simulink model "AN_Simulink_Model_v1_fil"  (R2019b)
settings: Solver=VariableStepAuto  StartTime=0.0  StopTime=testtime  RelTol=1e-3
InitFcn:
  | AN_InitFcn_Callback
StopFcn:
  | AN_StopFcn_Callback
values from neighbouring files (symbols this model uses):
  tdres = 1/Fs    (= 2.08333333333e-05)    [AN_Set_Model_Parameters.m]
libraries: hdlmdlgenlib x163, simulink x4, fillib x1, dspsrcs4 x1
(part 2 of 5)

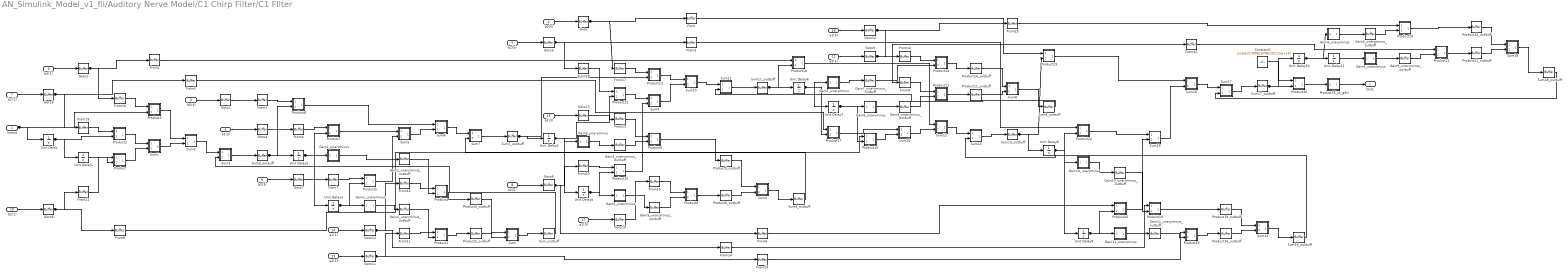
== system AN_Simulink_Model_v1_fil/Auditory Nerve Model/C1 Chirp Filter/C1 FIlter ==
  meout : Inport  OutDataTypeStr=single  PortDimensions=1  SampleTime=2.08333333333333e-05
  b0(5) : Inport  Port=2  OutDataTypeStr=single  PortDimensions=1  SampleTime=2.08333333333333e-05
  b0(3) : Inport  Port=3  OutDataTypeStr=single  PortDimensions=1  SampleTime=2.08333333333333e-05
  b0(1) : Inport  Port=4  OutDataTypeStr=single  PortDimensions=1  SampleTime=2.08333333333333e-05
  b1(5) : Inport  Port=5  OutDataTypeStr=single  PortDimensions=1  SampleTime=2.08333333333333e-05
  b1(3) : Inport  Port=6  OutDataTypeStr=single  PortDimensions=1  SampleTime=2.08333333333333e-05
  b1(1) : Inport  Port=7  OutDataTypeStr=single  PortDimensions=1  SampleTime=2.08333333333333e-05
  b2(5) : Inport  Port=8  OutDataTypeStr=single  PortDimensions=1  SampleTime=2.08333333333333e-05
  b2(3) : Inport  Port=9  OutDataTypeStr=single  PortDimensions=1  SampleTime=2.08333333333333e-05
  b2(1) : Inport  Port=10  OutDataTypeStr=single  PortDimensions=1  SampleTime=2.08333333333333e-05
  a2(5) : Inport  Port=11  OutDataTypeStr=single  PortDimensions=1  SampleTime=2.08333333333333e-05
  a2(3) : Inport  Port=12  OutDataTypeStr=single  PortDimensions=1  SampleTime=2.08333333333333e-05
  a2(1) : Inport  Port=13  OutDataTypeStr=single  PortDimensions=1  SampleTime=2.08333333333333e-05
  a1(1) : Inport  Port=14  OutDataTypeStr=single  PortDimensions=1  SampleTime=2.08333333333333e-05
  a1(3) : Inport  Port=15  OutDataTypeStr=single  PortDimensions=1  SampleTime=2.08333333333333e-05
  a1(5) : Inport  Port=16  OutDataTypeStr=single  PortDimensions=1  SampleTime=2.08333333333333e-05
  Constant1 : Constant  Value=single(3.398816786232115e+16)  OutDataTypeStr=single  SampleTime=-1
  From{,1..14,16..25} (25 alike) : hdlmdlgenlib/Buffer
      settings: SourceProductName=Simulink  SourceProductBaseCode=SL
  Gain10_unaryminus : Subsystem
      mask Display: disp('NFP\numinus');
  Gain10_unaryminus_outbuff : hdlmdlgenlib/Buffer
      settings: SourceProductName=Simulink  SourceProductBaseCode=SL
  Gain11_unaryminus : Subsystem
      mask Display: disp('NFP\numinus');
  Gain11_unaryminus_outbuff : hdlmdlgenlib/Buffer
      settings: SourceProductName=Simulink  SourceProductBaseCode=SL
  Gain1_unaryminus : Subsystem
      mask Display: disp('NFP\numinus');
  Gain1_unaryminus_outbuff : hdlmdlgenlib/Buffer
      settings: SourceProductName=Simulink  SourceProductBaseCode=SL
  Gain2_unaryminus : Subsystem
      mask Display: disp('NFP\numinus');
  Gain2_unaryminus_outbuff : hdlmdlgenlib/Buffer
      settings: SourceProductName=Simulink  SourceProductBaseCode=SL
  Gain3_unaryminus : Subsystem
      mask Display: disp('NFP\numinus');
  Gain3_unaryminus_outbuff : hdlmdlgenlib/Buffer
      settings: SourceProductName=Simulink  SourceProductBaseCode=SL
  Gain4_unaryminus : Subsystem
      mask Display: disp('NFP\numinus');
  Gain4_unaryminus_outbuff : hdlmdlgenlib/Buffer
      settings: SourceProductName=Simulink  SourceProductBaseCode=SL
  Gain5_unaryminus : Subsystem
      mask Display: disp('NFP\numinus');
  Gain5_unaryminus_outbuff : hdlmdlgenlib/Buffer
      settings: SourceProductName=Simulink  SourceProductBaseCode=SL
  Gain7_unaryminus : Subsystem
      mask Display: disp('NFP\numinus');
  Gain7_unaryminus_outbuff : hdlmdlgenlib/Buffer
      settings: SourceProductName=Simulink  SourceProductBaseCode=SL
  Gain8_unaryminus : Subsystem
      mask Display: disp('NFP\numinus');
  Gain8_unaryminus_outbuff : hdlmdlgenlib/Buffer
      settings: SourceProductName=Simulink  SourceProductBaseCode=SL
  Gain9_unaryminus : Subsystem
      mask Display: disp('NFP\numinus');
  Gain9_unaryminus_outbuff : hdlmdlgenlib/Buffer
      settings: SourceProductName=Simulink  SourceProductBaseCode=SL
  Goto{,1..14} (15 alike) : hdlmdlgenlib/Buffer
      settings: SourceProductName=Simulink  SourceProductBaseCode=SL
  Product : Subsystem
      mask Display: disp('NFP\nmul');
  Product1 : Subsystem
      mask Display: disp('NFP\nmul');
  Product10 : Subsystem
      mask Display: disp('NFP\nmul');
  Product11 : Subsystem
      mask Display: disp('NFP\nmul');
  Product11_outbuff : hdlmdlgenlib/Buffer
      settings: SourceProductName=Simulink  SourceProductBaseCode=SL
  Product12 : Subsystem
      mask Display: disp('NFP\nmul');
  Product13 : Subsystem
      mask Display: disp('NFP\nmul');
  Product14 : Subsystem
      mask Display: disp('NFP\nmul');
  Product14_outbuff : hdlmdlgenlib/Buffer
      settings: SourceProductName=Simulink  SourceProductBaseCode=SL
  Product15 : Subsystem
      mask Display: disp('NFP\nmul');
  Product16 : Subsystem
      mask Display: disp('NFP\nmul');
  Product16_outbuff : hdlmdlgenlib/Buffer
      settings: SourceProductName=Simulink  SourceProductBaseCode=SL
  Product17 : Subsystem
      mask Display: disp('NFP\nmul');
  Product18 : Subsystem
      mask Display: disp('NFP\nmul');
  Product19 : Subsystem
      mask Display: disp('NFP\nmul');
  Product19_outbuff : hdlmdlgenlib/Buffer
      settings: SourceProductName=Simulink  SourceProductBaseCode=SL
  Product1_outbuff : hdlmdlgenlib/Buffer
      settings: SourceProductName=Simulink  SourceProductBaseCode=SL
  Product2 : Subsystem
      mask Display: disp('NFP\nmul');
  Product20 : Subsystem
      mask Display: disp('NFP\nmul');
  Product21 : Subsystem
      mask Display: disp('NFP\nmul');
  Product21_outbuff : hdlmdlgenlib/Buffer
      settings: SourceProductName=Simulink  SourceProductBaseCode=SL
  Product22 : Subsystem
      mask Display: disp('NFP\nmul');
  Product23 : Subsystem
      mask Display: disp('NFP\nmul');
  Product24 : Subsystem
      mask Display: disp('NFP\nmul');
  Product24_outbuff : hdlmdlgenlib/Buffer
      settings: SourceProductName=Simulink  SourceProductBaseCode=SL
  Product25_to_gain : Subsystem
      mask Display: disp('NFP\ngain_pow2');
  Product26 : Subsystem
      mask Display: disp('NFP\nmul');
  Product3 : Subsystem
      mask Display: disp('NFP\nmul');
  Product4 : Subsystem
      mask Display: disp('NFP\nmul');
  Product4_outbuff : hdlmdlgenlib/Buffer
      settings: SourceProductName=Simulink  SourceProductBaseCode=SL
  Product5 : Subsystem
      mask Display: disp('NFP\nmul');
  Product6 : Subsystem
      mask Display: disp('NFP\nmul');
  Product6_outbuff : hdlmdlgenlib/Buffer
      settings: SourceProductName=Simulink  SourceProductBaseCode=SL
  Product7 : Subsystem
      mask Display: disp('NFP\nmul');
  Product8 : Subsystem
      mask Display: disp('NFP\nmul');
  Product9 : Subsystem
      mask Display: disp('NFP\nmul');
  Product9_outbuff : hdlmdlgenlib/Buffer
      settings: SourceProductName=Simulink  SourceProductBaseCode=SL
  Sum : Subsystem
      mask Display: disp('NFP\nadd');
  Sum1 : Subsystem
      mask Display: disp('NFP\nadd');
  Sum10 : Subsystem
      mask Display: disp('NFP\nadd');
  Sum11 : Subsystem
      mask Display: disp('NFP\nadd');
  Sum11_outbuff : hdlmdlgenlib/Buffer
      settings: SourceProductName=Simulink  SourceProductBaseCode=SL
  Sum12 : Subsystem
      mask Display: disp('NFP\nadd');
  Sum13 : Subsystem
      mask Display: disp('NFP\nadd');
  Sum13_outbuff : hdlmdlgenlib/Buffer
      settings: SourceProductName=Simulink  SourceProductBaseCode=SL
  Sum14 : Subsystem
      mask Display: disp('NFP\nadd');
  Sum14_outbuff : hdlmdlgenlib/Buffer
      settings: SourceProductName=Simulink  SourceProductBaseCode=SL
  Sum15 : Subsystem
      mask Display: disp('NFP\nadd');
  Sum16 : Subsystem
      mask Display: disp('NFP\nadd');
  Sum17 : Subsystem
      mask Display: disp('NFP\nadd');
  Sum17_outbuff : hdlmdlgenlib/Buffer
      settings: SourceProductName=Simulink  SourceProductBaseCode=SL
  Sum18 : Subsystem
      mask Display: disp('NFP\nadd');
  Sum18_outbuff : hdlmdlgenlib/Buffer
      settings: SourceProductName=Simulink  SourceProductBaseCode=SL
  Sum19 : Subsystem
      mask Display: disp('NFP\nadd');
  Sum2 : Subsystem
      mask Display: disp('NFP\nadd');
  Sum3 : Subsystem
      mask Display: disp('NFP\nadd');
  Sum3_outbuff : hdlmdlgenlib/Buffer
      settings: SourceProductName=Simulink  SourceProductBaseCode=SL
  Sum4 : Subsystem
      mask Display: disp('NFP\nadd');
  Sum4_outbuff : hdlmdlgenlib/Buffer
      settings: SourceProductName=Simulink  SourceProductBaseCode=SL
  Sum5 : Subsystem
      mask Display: disp('NFP\nadd');
  Sum6 : Subsystem
      mask Display: disp('NFP\nadd');
  Sum7 : Subsystem
      mask Display: disp('NFP\nadd');
  Sum7_outbuff : hdlmdlgenlib/Buffer
      settings: SourceProductName=Simulink  SourceProductBaseCode=SL
  Sum8 : Subsystem
      mask Display: disp('NFP\nadd');
  Sum8_outbuff : hdlmdlgenlib/Buffer
      settings: SourceProductName=Simulink  SourceProductBaseCode=SL
  Sum9 : Subsystem
      mask Display: disp('NFP\nadd');
  Sum_outbuff : hdlmdlgenlib/Buffer
      settings: SourceProductName=Simulink  SourceProductBaseCode=SL
  Unit Delay{,1..11} (12 alike) : UnitDelay  InitialCondition=single(0)  SampleTime=2.08333333333333e-05
  Out1 : Outport  VectorParamsAs1DForOutWhenUnconnected=off
  wires:
  Product25_to_gain/1(Out1) -> Out1/1
  Sum9/1(Out1) -> Sum10/2(In2)
  Sum8/1(Out1) -> Sum8_outbuff/1
  Sum7/1(Out1) -> Sum7_outbuff/1
  Sum6/1(Out1) -> Sum7/1(In1)
  Sum5/1(Out1) -> Sum6/2(In2)
  Sum4/1(Out1) -> Sum4_outbuff/1
  Sum3/1(Out1) -> Sum3_outbuff/1
  Sum2/1(Out1) -> Sum3/1(In1)
  Sum19/1(Out1) -> Sum16/2(In2)
  Sum18/1(Out1) -> Sum18_outbuff/1
  Sum17/1(Out1) -> Sum17_outbuff/1
  Sum16/1(Out1) -> Sum17/1(In1)
  Sum15/1(Out1) -> Sum12/2(In2)
  Sum14/1(Out1) -> Sum14_outbuff/1
  Sum13/1(Out1) -> Sum13_outbuff/1
  Sum12/1(Out1) -> Sum13/1(In1)
  Sum11/1(Out1) -> Sum11_outbuff/1
  Sum10/1(Out1) -> Sum11/1(In1)
  Sum1/1(Out1) -> Sum2/2(In2)
  Sum/1(Out1) -> Sum_outbuff/1
  Product9/1(Out1) -> Product9_outbuff/1
  Product8/1(Out1) -> Sum6/1(In1)
  Product7/1(Out1) -> Sum5/1(In1)
  Product6/1(Out1) -> Product6_outbuff/1
  Product5/1(Out1) -> Sum5/2(In2)
  Product4/1(Out1) -> Product4_outbuff/1
  Product3/1(Out1) -> Sum2/1(In1)
  Product26/1(Out1) -> Product25_to_gain/1(In1)
  Product24/1(Out1) -> Product24_outbuff/1
  Product23/1(Out1) -> Sum16/1(In1)
  Product22/1(Out1) -> Sum19/1(In1)
  Product21/1(Out1) -> Product21_outbuff/1
  Product20/1(Out1) -> Sum19/2(In2)
  Product2/1(Out1) -> Sum1/1(In1)
  Product19/1(Out1) -> Product19_outbuff/1
  Product18/1(Out1) -> Sum12/1(In1)
  Product17/1(Out1) -> Sum15/1(In1)
  Product16/1(Out1) -> Product16_outbuff/1
  Product15/1(Out1) -> Sum15/2(In2)
  Product14/1(Out1) -> Product14_outbuff/1
  Product13/1(Out1) -> Sum10/1(In1)
  Product12/1(Out1) -> Sum9/1(In1)
  Product11/1(Out1) -> Product11_outbuff/1
  Product10/1(Out1) -> Sum9/2(In2)
  Product1/1(Out1) -> Product1_outbuff/1
  Product/1(Out1) -> Sum1/2(In2)
  Gain9_unaryminus/1(Out1) -> Gain9_unaryminus_outbuff/1
  Gain8_unaryminus/1(Out1) -> Gain8_unaryminus_outbuff/1
  Gain7_unaryminus/1(Out1) -> Gain7_unaryminus_outbuff/1
  Gain5_unaryminus/1(Out1) -> Gain5_unaryminus_outbuff/1
  Gain4_unaryminus/1(Out1) -> Gain4_unaryminus_outbuff/1
  Gain3_unaryminus/1(Out1) -> Gain3_unaryminus_outbuff/1
  Gain2_unaryminus/1(Out1) -> Gain2_unaryminus_outbuff/1
  Gain11_unaryminus/1(Out1) -> Gain11_unaryminus_outbuff/1
  Gain10_unaryminus/1(Out1) -> Gain10_unaryminus_outbuff/1
  Gain1_unaryminus/1(Out1) -> Gain1_unaryminus_outbuff/1
  Goto7/1 -> From7/1
  Goto4/1 -> From4/1
  Goto9/1 -> From22/1, From9/1
  Goto8/1 -> From21/1, From8/1
  Goto6/1 -> From20/1, From6/1
  Goto5/1 -> From19/1, From5/1
  Goto3/1 -> From18/1, From3/1
  Goto2/1 -> From16/1, From2/1
  Goto14/1 -> From14/1, From25/1
  Goto13/1 -> From13/1
  Goto12/1 -> From12/1, From24/1
  Goto11/1 -> From11/1, From23/1
  Goto10/1 -> From10/1
  Goto1/1 -> From1/1
  Goto/1 -> From/1, From17/1
  Unit Delay9/1 -> Gain11_unaryminus/1(In1), Product20/2(In2)
  Unit Delay8/1 -> Unit Delay9/1, Gain10_unaryminus/1(In1), Product22/2(In2)
  Unit Delay7/1 -> Gain8_unaryminus/1(In1), Product15/2(In2)
  Unit Delay6/1 -> Unit Delay7/1, Gain7_unaryminus/1(In1), Product17/2(In2)
  Unit Delay5/1 -> Gain5_unaryminus/1(In1), Product10/2(In2)
  Unit Delay4/1 -> Unit Delay5/1, Gain3_unaryminus/1(In1), Product12/2(In2)
  Unit Delay3/1 -> Gain2_unaryminus/1(In1), Product5/2(In2)
  Unit Delay2/1 -> Unit Delay3/1, Gain1_unaryminus/1(In1), Product7/2(In2)
  Unit Delay11/1 -> Gain9_unaryminus/1(In1)
  Unit Delay10/1 -> Unit Delay11/1, Gain4_unaryminus/1(In1)
  Unit Delay1/1 -> Product/2(In2)
  Unit Delay/1 -> Unit Delay1/1, Product2/2(In2)
  Sum8_outbuff/1 -> Sum11/2(In2)
  Sum7_outbuff/1 -> Unit Delay4/1, Product13/2(In2)
  Sum4_outbuff/1 -> Sum7/2(In2)
  Sum3_outbuff/1 -> Unit Delay2/1, Product8/2(In2)
  Sum18_outbuff/1 -> Sum17/2(In2)
  Sum17_outbuff/1 -> Unit Delay10/1, Product26/2(In2)
  Sum14_outbuff/1 -> Sum13/2(In2)
  Sum13_outbuff/1 -> Unit Delay8/1, Product23/2(In2)
  Sum11_outbuff/1 -> Unit Delay6/1, Product18/2(In2)
  Sum_outbuff/1 -> Sum3/2(In2)
  Product9_outbuff/1 -> Sum4/1(In1)
  Product6_outbuff/1 -> Sum4/2(In2)
  Product4_outbuff/1 -> Sum/1(In1)
  Product24_outbuff/1 -> Sum18/1(In1)
  Product21_outbuff/1 -> Sum18/2(In2)
  Product19_outbuff/1 -> Sum14/1(In1)
  Product16_outbuff/1 -> Sum14/2(In2)
  Product14_outbuff/1 -> Sum8/1(In1)
  Product11_outbuff/1 -> Sum8/2(In2)
  Product1_outbuff/1 -> Sum/2(In2)
  Gain9_unaryminus_outbuff/1 -> Product21/2(In2)
  Gain8_unaryminus_outbuff/1 -> Product11/2(In2)
  Gain7_unaryminus_outbuff/1 -> Product14/2(In2)
  Gain5_unaryminus_outbuff/1 -> Product6/2(In2)
  Gain4_unaryminus_outbuff/1 -> Product24/2(In2)
  Gain3_unaryminus_outbuff/1 -> Product9/2(In2)
  Gain2_unaryminus_outbuff/1 -> Product1/2(In2)
  Gain11_unaryminus_outbuff/1 -> Product16/2(In2)
  Gain10_unaryminus_outbuff/1 -> Product19/2(In2)
  Gain1_unaryminus_outbuff/1 -> Product4/2(In2)
  From9/1 -> Product11/1(In1)
  From8/1 -> Product15/1(In1)
  From7/1 -> Product5/1(In1)
  From6/1 -> Product20/1(In1)
  From5/1 -> Product17/1(In1)
  From4/1 -> Product7/1(In1)
  From3/1 -> Product22/1(In1)
  From25/1 -> Product24/1(In1)
  From24/1 -> Product19/1(In1)
  From23/1 -> Product16/1(In1)
  From22/1 -> Product21/1(In1)
  From21/1 -> Product/1(In1)
  From20/1 -> Product10/1(In1)
  From2/1 -> Product18/1(In1)
  From19/1 -> Product2/1(In1)
  From18/1 -> Product12/1(In1)
  From17/1 -> Product13/1(In1)
  From16/1 -> Product3/1(In1)
  From14/1 -> Product14/1(In1)
  From13/1 -> Product9/1(In1)
  From12/1 -> Product4/1(In1)
  From11/1 -> Product1/1(In1)
  From10/1 -> Product6/1(In1)
  From1/1 -> Product8/1(In1)
  From/1 -> Product23/1(In1)
  Constant1/1 -> Product26/1(In1)
  a1(5)/1 -> Goto14/1
  a1(3)/1 -> Goto13/1
  a1(1)/1 -> Goto12/1
  a2(1)/1 -> Goto11/1
  a2(3)/1 -> Goto10/1
  a2(5)/1 -> Goto9/1
  b2(1)/1 -> Goto8/1
  b2(3)/1 -> Goto7/1
  b2(5)/1 -> Goto6/1
  b1(1)/1 -> Goto5/1
  b1(3)/1 -> Goto4/1
  b1(5)/1 -> Goto3/1
  b0(1)/1 -> Goto2/1
  b0(3)/1 -> Goto1/1
  b0(5)/1 -> Goto/1
  meout/1 -> Unit Delay/1, Product3/2(In2)

== system AN_Simulink_Model_v1_fil/Auditory Nerve Model/C1 Chirp Filter/Calculate C1filterout ==
  C1filterouttmp : Inport  OutDataTypeStr=single  PortDimensions=1  SampleTime=2.08333333333333e-05
  Gain1_unary : hdlmdlgenlib/Buffer
      settings: SourceProductName=Simulink  SourceProductBaseCode=SL
  C1filterout : Outport  VectorParamsAs1DForOutWhenUnconnected=off
  wires:
  Gain1_unary/1 -> C1filterout/1
  C1filterouttmp/1 -> Gain1_unary/1

== system AN_Simulink_Model_v1_fil/Auditory Nerve Model/C1 Chirp Filter/Calculate rsigma ==
  tauc1 : Inport  OutDataTypeStr=single  PortDimensions=1  SampleTime=2.08333333333333e-05
  Constant2 : Constant  Value=single(0.003011211520060897)  OutDataTypeStr=single  SampleTime=-1
  Reciprocal1_recip : Subsystem
      mask Display: disp('NFP\nmath');
  Reciprocal_recip : Subsystem
      mask Display: disp('NFP\nmath');
  Subtract : Subsystem
      mask Display: disp('NFP\nadd');
  rsigma : Outport  VectorParamsAs1DForOutWhenUnconnected=off
  wires:
  Subtract/1(Out1) -> rsigma/1
  Reciprocal1_recip/1(Out1) -> Subtract/2(In2)
  Reciprocal_recip/1(Out1) -> Subtract/1(In1)
  Constant2/1 -> Reciprocal1_recip/1(In1)
  tauc1/1 -> Reciprocal_recip/1(In1)

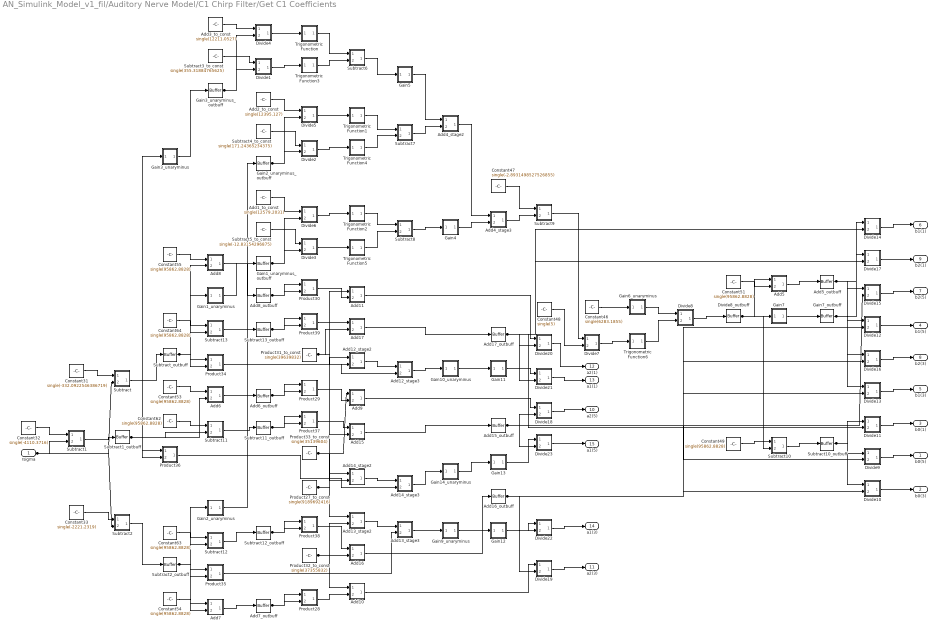
== system AN_Simulink_Model_v1_fil/Auditory Nerve Model/C1 Chirp Filter/Get C1 Coefficients ==
  rsigma : Inport  OutDataTypeStr=single  PortDimensions=1  SampleTime=2.08333333333333e-05
  Add10 : Subsystem
      mask Display: disp('NFP\nadd');
  Add11 : Subsystem
      mask Display: disp('NFP\nadd');
  Add12_stage2 : Subsystem
      mask Display: disp('NFP\nadd');
  Add12_stage3 : Subsystem
      mask Display: disp('NFP\nadd');
  Add13_stage2 : Subsystem
      mask Display: disp('NFP\nadd');
  Add13_stage3 : Subsystem
      mask Display: disp('NFP\nadd');
  Add14_stage2 : Subsystem
      mask Display: disp('NFP\nadd');
  Add14_stage3 : Subsystem
      mask Display: disp('NFP\nadd');
  Add15 : Subsystem
      mask Display: disp('NFP\nadd');
  Add15_outbuff : hdlmdlgenlib/Buffer
      settings: SourceProductName=Simulink  SourceProductBaseCode=SL
  Add16 : Subsystem
      mask Display: disp('NFP\nadd');
  Add16_outbuff : hdlmdlgenlib/Buffer
      settings: SourceProductName=Simulink  SourceProductBaseCode=SL
  Add17 : Subsystem
      mask Display: disp('NFP\nadd');
  Add17_outbuff : hdlmdlgenlib/Buffer
      settings: SourceProductName=Simulink  SourceProductBaseCode=SL
  Add1_to_const : Constant  Value=single(12579.2031)  OutDataTypeStr=single  SampleTime=-1
  Add2_to_const : Constant  Value=single(12395.127)  OutDataTypeStr=single  SampleTime=-1
  Add3_to_const : Constant  Value=single(12211.0527)  OutDataTypeStr=single  SampleTime=-1
  Add4_stage2 : Subsystem
      mask Display: disp('NFP\nadd');
  Add4_stage3 : Subsystem
      mask Display: disp('NFP\nadd');
  Add5 : Subsystem
      mask Display: disp('NFP\nadd');
  Add5_outbuff : hdlmdlgenlib/Buffer
      settings: SourceProductName=Simulink  SourceProductBaseCode=SL
  Add6 : Subsystem
      mask Display: disp('NFP\nadd');
  Add6_outbuff : hdlmdlgenlib/Buffer
      settings: SourceProductName=Simulink  SourceProductBaseCode=SL
  Add7 : Subsystem
      mask Display: disp('NFP\nadd');
  Add7_outbuff : hdlmdlgenlib/Buffer
      settings: SourceProductName=Simulink  SourceProductBaseCode=SL
  Add8 : Subsystem
      mask Display: disp('NFP\nadd');
  Add8_outbuff : hdlmdlgenlib/Buffer
      settings: SourceProductName=Simulink  SourceProductBaseCode=SL
  Add9 : Subsystem
      mask Display: disp('NFP\nadd');
  Constant31 : Constant  Value=single(-332.0922546386719)  OutDataTypeStr=single  SampleTime=-1
  Constant32 : Constant  Value=single(-4110.3716)  OutDataTypeStr=single  SampleTime=-1
  Constant33 : Constant  Value=single(-2221.2319)  OutDataTypeStr=single  SampleTime=-1
  Constant46 : Constant  Value=single(6283.1855)  OutDataTypeStr=single  SampleTime=-1
  Constant47 : Constant  Value=single(-2.8931498527526855)  OutDataTypeStr=single  SampleTime=-1
  Constant48 : Constant  Value=single(5)  OutDataTypeStr=single  SampleTime=-1
  Constant{49,51,53..55,62..64} (8 alike) : Constant  Value=single(95862.8828)  OutDataTypeStr=single  SampleTime=-1
  Divide1 : Subsystem
      mask Display: disp('NFP\nmul');
  Divide10 : Subsystem
      mask Display: disp('NFP\nmul');
  Divide11 : Subsystem
      mask Display: disp('NFP\nmul');
  Divide12 : Subsystem
      mask Display: disp('NFP\nmul');
  Divide13 : Subsystem
      mask Display: disp('NFP\nmul');
  Divide14 : Subsystem
      mask Display: disp('NFP\nmul');
  Divide15 : Subsystem
      mask Display: disp('NFP\nmul');
  Divide16 : Subsystem
      mask Display: disp('NFP\nmul');
  Divide17 : Subsystem
      mask Display: disp('NFP\nmul');
  Divide18 : Subsystem
      mask Display: disp('NFP\nmul');
  Divide19 : Subsystem
      mask Display: disp('NFP\nmul');
  Divide2 : Subsystem
      mask Display: disp('NFP\nmul');
  Divide20 : Subsystem
      mask Display: disp('NFP\nmul');
  Divide21 : Subsystem
      mask Display: disp('NFP\nmul');
  Divide22 : Subsystem
      mask Display: disp('NFP\nmul');
  Divide23 : Subsystem
      mask Display: disp('NFP\nmul');
  Divide3 : Subsystem
      mask Display: disp('NFP\nmul');
  Divide4 : Subsystem
      mask Display: disp('NFP\nmul');
  Divide5 : Subsystem
      mask Display: disp('NFP\nmul');
  Divide6 : Subsystem
      mask Display: disp('NFP\nmul');
  Divide7 : Subsystem
      mask Display: disp('NFP\nmul');
  Divide8 : Subsystem
      mask Display: disp('NFP\nmul');
  Divide8_outbuff : hdlmdlgenlib/Buffer
      settings: SourceProductName=Simulink  SourceProductBaseCode=SL
  Divide9 : Subsystem
      mask Display: disp('NFP\nmul');
  Gain10_unaryminus : Subsystem
      mask Display: disp('NFP\numinus');
  Gain11 : Subsystem
      mask Display: disp('NFP\ngain_pow2');
  Gain12 : Subsystem
      mask Display: disp('NFP\ngain_pow2');
  Gain13 : Subsystem
      mask Display: disp('NFP\ngain_pow2');
  Gain14_unaryminus : Subsystem
      mask Display: disp('NFP\numinus');
  Gain1_unaryminus : Subsystem
      mask Display: disp('NFP\numinus');
  Gain1_unaryminus_outbuff : hdlmdlgenlib/Buffer
      settings: SourceProductName=Simulink  SourceProductBaseCode=SL
  Gain2_unaryminus : Subsystem
      mask Display: disp('NFP\numinus');
  Gain2_unaryminus_outbuff : hdlmdlgenlib/Buffer
      settings: SourceProductName=Simulink  SourceProductBaseCode=SL
  Gain3_unaryminus : Subsystem
      mask Display: disp('NFP\numinus');
  Gain3_unaryminus_outbuff : hdlmdlgenlib/Buffer
      settings: SourceProductName=Simulink  SourceProductBaseCode=SL
  Gain4 : Subsystem
      mask Display: disp('NFP\ngain_pow2');
  Gain5 : Subsystem
      mask Display: disp('NFP\ngain_pow2');
  Gain6_unaryminus : Subsystem
      mask Display: disp('NFP\numinus');
  Gain7 : Subsystem
      mask Display: disp('NFP\ngain_pow2');
  Gain7_outbuff : hdlmdlgenlib/Buffer
      settings: SourceProductName=Simulink  SourceProductBaseCode=SL
  Gain9_unaryminus : Subsystem
      mask Display: disp('NFP\numinus');
  Product27_to_const : Constant  Value=single(9189692416)  OutDataTypeStr=single  SampleTime=-1
  Product28 : Subsystem
      mask Display: disp('NFP\nmul');
  Product29 : Subsystem
      mask Display: disp('NFP\nmul');
  Product30 : Subsystem
      mask Display: disp('NFP\nmul');
  Product31_to_const : Constant  Value=single(39639832)  OutDataTypeStr=single  SampleTime=-1
  Product32_to_const : Constant  Value=single(37355832)  OutDataTypeStr=single  SampleTime=-1
  Product33_to_const : Constant  Value=single(35139604)  OutDataTypeStr=single  SampleTime=-1
  Product34 : Subsystem
      mask Display: disp('NFP\nmul');
  Product35 : Subsystem
      mask Display: disp('NFP\nmul');
  Product36 : Subsystem
      mask Display: disp('NFP\nmul');
  Product37 : Subsystem
      mask Display: disp('NFP\nmul');
  Product38 : Subsystem
      mask Display: disp('NFP\nmul');
  Product39 : Subsystem
      mask Display: disp('NFP\nmul');
  Subtract : Subsystem
      mask Display: disp('NFP\nadd');
  Subtract1 : Subsystem
      mask Display: disp('NFP\nadd');
  Subtract10 : Subsystem
      mask Display: disp('NFP\nadd');
  Subtract10_outbuff : hdlmdlgenlib/Buffer
      settings: SourceProductName=Simulink  SourceProductBaseCode=SL
  Subtract11 : Subsystem
      mask Display: disp('NFP\nadd');
  Subtract11_outbuff : hdlmdlgenlib/Buffer
      settings: SourceProductName=Simulink  SourceProductBaseCode=SL
  Subtract12 : Subsystem
      mask Display: disp('NFP\nadd');
  Subtract12_outbuff : hdlmdlgenlib/Buffer
      settings: SourceProductName=Simulink  SourceProductBaseCode=SL
  Subtract13 : Subsystem
      mask Display: disp('NFP\nadd');
  Subtract13_outbuff : hdlmdlgenlib/Buffer
      settings: SourceProductName=Simulink  SourceProductBaseCode=SL
  Subtract1_outbuff : hdlmdlgenlib/Buffer
      settings: SourceProductName=Simulink  SourceProductBaseCode=SL
  Subtract2 : Subsystem
      mask Display: disp('NFP\nadd');
  Subtract2_outbuff : hdlmdlgenlib/Buffer
      settings: SourceProductName=Simulink  SourceProductBaseCode=SL
  Subtract3_to_const : Constant  Value=single(355.31884765625)  OutDataTypeStr=single  SampleTime=-1
  Subtract4_to_const : Constant  Value=single(171.24365234375)  OutDataTypeStr=single  SampleTime=-1
  Subtract5_to_const : Constant  Value=single(-12.83154296875)  OutDataTypeStr=single  SampleTime=-1
  Subtract6 : Subsystem
      mask Display: disp('NFP\nadd');
  Subtract7 : Subsystem
      mask Display: disp('NFP\nadd');
  Subtract8 : Subsystem
      mask Display: disp('NFP\nadd');
  Subtract9 : Subsystem
      mask Display: disp('NFP\nadd');
  Subtract_outbuff : hdlmdlgenlib/Buffer
      settings: SourceProductName=Simulink  SourceProductBaseCode=SL
  Trigonometric Function : Subsystem
      mask Display: disp('NFP\ntrig');
  Trigonometric Function1 : Subsystem
      mask Display: disp('NFP\ntrig');
  Trigonometric Function2 : Subsystem
      mask Display: disp('NFP\ntrig');
  Trigonometric Function3 : Subsystem
      mask Display: disp('NFP\ntrig');
  Trigonometric Function4 : Subsystem
      mask Display: disp('NFP\ntrig');
  Trigonometric Function5 : Subsystem
      mask Display: disp('NFP\ntrig');
  Trigonometric Function6 : Subsystem
      mask Display: disp('NFP\ntrig');
  b0(5) : Outport  VectorParamsAs1DForOutWhenUnconnected=off
  b0(3) : Outport  Port=2  VectorParamsAs1DForOutWhenUnconnected=off
  b0(1) : Outport  Port=3  VectorParamsAs1DForOutWhenUnconnected=off
  b1(5) : Outport  Port=4  VectorParamsAs1DForOutWhenUnconnected=off
  b1(3) : Outport  Port=5  VectorParamsAs1DForOutWhenUnconnected=off
  b1(1) : Outport  Port=6  VectorParamsAs1DForOutWhenUnconnected=off
  b2(5) : Outport  Port=7  VectorParamsAs1DForOutWhenUnconnected=off
  b2(3) : Outport  Port=8  VectorParamsAs1DForOutWhenUnconnected=off
  b2(1) : Outport  Port=9  VectorParamsAs1DForOutWhenUnconnected=off
  a2(5) : Outport  Port=10  VectorParamsAs1DForOutWhenUnconnected=off
  a2(3) : Outport  Port=11  VectorParamsAs1DForOutWhenUnconnected=off
  a2(1) : Outport  Port=12  VectorParamsAs1DForOutWhenUnconnected=off
  a1(1) : Outport  Port=13  VectorParamsAs1DForOutWhenUnconnected=off
  a1(3) : Outport  Port=14  VectorParamsAs1DForOutWhenUnconnected=off
  a1(5) : Outport  Port=15  VectorParamsAs1DForOutWhenUnconnected=off
  wires:
  Trigonometric Function6/1(Out1) -> Divide8/2(In2)
  Trigonometric Function5/1(Out1) -> Subtract8/2(In2)
  Trigonometric Function4/1(Out1) -> Subtract7/2(In2)
  Trigonometric Function3/1(Out1) -> Subtract6/2(In2)
  Trigonometric Function2/1(Out1) -> Subtract8/1(In1)
  Trigonometric Function1/1(Out1) -> Subtract7/1(In1)
  Trigonometric Function/1(Out1) -> Subtract6/1(In1)
  Subtract9/1(Out1) -> Divide7/1(In1)
  Subtract8/1(Out1) -> Gain4/1(In1)
  Subtract7/1(Out1) -> Add4_stage2/2(In2)
  Subtract6/1(Out1) -> Gain5/1(In1)
  Subtract2/1(Out1) -> Subtract2_outbuff/1
  Subtract13/1(Out1) -> Subtract13_outbuff/1
  Subtract12/1(Out1) -> Subtract12_outbuff/1
  Subtract11/1(Out1) -> Subtract11_outbuff/1
  Subtract10/1(Out1) -> Subtract10_outbuff/1
  Subtract1/1(Out1) -> Subtract1_outbuff/1
  Subtract/1(Out1) -> Subtract_outbuff/1
  Product39/1(Out1) -> Add17/1(In1)
  Product38/1(Out1) -> Add16/1(In1)
  Product37/1(Out1) -> Add15/1(In1)
  Product36/1(Out1) -> Add14_stage3/2(In2)
  Product35/1(Out1) -> Add13_stage3/2(In2)
  Product34/1(Out1) -> Add12_stage3/2(In2)
  Product30/1(Out1) -> Add11/2(In2)
  Product29/1(Out1) -> Add9/2(In2)
  Product28/1(Out1) -> Add10/2(In2)
  Divide9/1(Out1) -> b0(5)/1
  Divide8/1(Out1) -> Divide8_outbuff/1
  Divide7/1(Out1) -> Trigonometric Function6/1(In1)
  Divide6/1(Out1) -> Trigonometric Function2/1(In1)
  Divide5/1(Out1) -> Trigonometric Function1/1(In1)
  Divide4/1(Out1) -> Trigonometric Function/1(In1)
  Divide3/1(Out1) -> Trigonometric Function5/1(In1)
  Divide23/1(Out1) -> a1(5)/1
  Divide22/1(Out1) -> a1(3)/1
  Divide21/1(Out1) -> a1(1)/1
  Divide20/1(Out1) -> a2(1)/1
  Divide2/1(Out1) -> Trigonometric Function4/1(In1)
  Divide19/1(Out1) -> a2(3)/1
  Divide18/1(Out1) -> a2(5)/1
  Divide17/1(Out1) -> b2(1)/1
  Divide16/1(Out1) -> b2(3)/1
  Divide15/1(Out1) -> b2(5)/1
  Divide14/1(Out1) -> b1(1)/1
  Divide13/1(Out1) -> b1(3)/1
  Divide12/1(Out1) -> b1(5)/1
  Divide11/1(Out1) -> b0(1)/1
  Divide10/1(Out1) -> b0(3)/1
  Divide1/1(Out1) -> Trigonometric Function3/1(In1)
  Add9/1(Out1) -> Divide18/1(In1)
  Add8/1(Out1) -> Add8_outbuff/1
  Add7/1(Out1) -> Add7_outbuff/1
  Add6/1(Out1) -> Add6_outbuff/1
  Add5/1(Out1) -> Add5_outbuff/1
  Add4_stage3/1(Out1) -> Subtract9/2(In2)
  Add4_stage2/1(Out1) -> Add4_stage3/1(In1)
  Add17/1(Out1) -> Add17_outbuff/1
  Add16/1(Out1) -> Add16_outbuff/1
  Add15/1(Out1) -> Add15_outbuff/1
  Add14_stage3/1(Out1) -> Gain14_unaryminus/1(In1)
  Add14_stage2/1(Out1) -> Add14_stage3/1(In1)
  Add13_stage3/1(Out1) -> Gain9_unaryminus/1(In1)
  Add13_stage2/1(Out1) -> Add13_stage3/1(In1)
  Add12_stage3/1(Out1) -> Gain10_unaryminus/1(In1)
  Add12_stage2/1(Out1) -> Add12_stage3/1(In1)
  Add11/1(Out1) -> Divide20/1(In1)
  Add10/1(Out1) -> Divide19/1(In1)
  Gain9_unaryminus/1(Out1) -> Gain12/1(In1)
  Gain7/1(Out1) -> Gain7_outbuff/1
  Gain6_unaryminus/1(Out1) -> Divide8/1(In1)
  Gain5/1(Out1) -> Add4_stage2/1(In1)
  Gain4/1(Out1) -> Add4_stage3/2(In2)
  Gain3_unaryminus/1(Out1) -> Gain3_unaryminus_outbuff/1
  Gain2_unaryminus/1(Out1) -> Gain2_unaryminus_outbuff/1
  Gain14_unaryminus/1(Out1) -> Gain13/1(In1)
  Gain13/1(Out1) -> Divide23/1(In1)
  Gain12/1(Out1) -> Divide22/1(In1)
  Gain11/1(Out1) -> Divide21/1(In1)
  Gain10_unaryminus/1(Out1) -> Gain11/1(In1)
  Gain1_unaryminus/1(Out1) -> Gain1_unaryminus_outbuff/1
  Subtract5_to_const/1 -> Divide3/1(In1)
  Subtract4_to_const/1 -> Divide2/1(In1)
  Subtract3_to_const/1 -> Divide1/1(In1)
  Subtract2_outbuff/1 -> Gain2_unaryminus/1(In1), Add7/2(In2), Product35/1(In1), Product35/2(In2), Subtract12/2(In2)
  Subtract13_outbuff/1 -> Product39/1(In1), Product39/2(In2)
  Subtract12_outbuff/1 -> Product38/1(In1), Product38/2(In2)
  Subtract11_outbuff/1 -> Product37/1(In1), Product37/2(In2)
  Subtract10_outbuff/1 -> Divide10/1(In1), Divide11/1(In1), Divide9/1(In1)
  Subtract1_outbuff/1 -> Gain3_unaryminus/1(In1), Add6/2(In2), Product36/1(In1), Product36/2(In2), Subtract11/2(In2)
  Subtract_outbuff/1 -> Gain1_unaryminus/1(In1), Add8/2(In2), Product34/1(In1), Product34/2(In2), Subtract13/2(In2)
  Product33_to_const/1 -> Add14_stage2/2(In2), Add15/2(In2), Add9/1(In1)
  Product32_to_const/1 -> Add10/1(In1), Add13_stage2/2(In2), Add16/2(In2)
  Product31_to_const/1 -> Add11/1(In1), Add12_stage2/2(In2), Add17/2(In2)
  Product27_to_const/1 -> Add12_stage2/1(In1), Add13_stage2/1(In1), Add14_stage2/1(In1)
  Gain7_outbuff/1 -> Divide12/1(In1), Divide13/1(In1), Divide14/1(In1)
  Gain3_unaryminus_outbuff/1 -> Divide1/2(In2), Divide4/2(In2)
  Gain2_unaryminus_outbuff/1 -> Divide2/2(In2), Divide5/2(In2)
  Gain1_unaryminus_outbuff/1 -> Divide3/2(In2), Divide6/2(In2)
  Divide8_outbuff/1 -> Gain7/1(In1), Add5/1(In1), Subtract10/2(In2)
  Constant64/1 -> Subtract13/1(In1)
  Constant63/1 -> Subtract12/1(In1)
  Constant62/1 -> Subtract11/1(In1)
  Constant55/1 -> Add8/1(In1)
  Constant54/1 -> Add7/1(In1)
  Constant53/1 -> Add6/1(In1)
  Constant51/1 -> Add5/2(In2)
  Constant49/1 -> Subtract10/1(In1)
  Constant48/1 -> Divide7/2(In2)
  Constant47/1 -> Subtract9/1(In1)
  Constant46/1 -> Gain6_unaryminus/1(In1)
  Constant33/1 -> Subtract2/1(In1)
  Constant32/1 -> Subtract1/1(In1)
  Constant31/1 -> Subtract/1(In1)
  Add8_outbuff/1 -> Product30/1(In1), Product30/2(In2)
  Add7_outbuff/1 -> Product28/1(In1), Product28/2(In2)
  Add6_outbuff/1 -> Product29/1(In1), Product29/2(In2)
  Add5_outbuff/1 -> Divide15/1(In1), Divide16/1(In1), Divide17/1(In1)
  Add3_to_const/1 -> Divide4/1(In1)
  Add2_to_const/1 -> Divide5/1(In1)
  Add17_outbuff/1 -> Divide11/2(In2), Divide14/2(In2), Divide17/2(In2), Divide20/2(In2), Divide21/2(In2)
  Add16_outbuff/1 -> Divide10/2(In2), Divide13/2(In2), Divide16/2(In2), Divide19/2(In2), Divide22/2(In2)
  Add15_outbuff/1 -> Divide12/2(In2), Divide15/2(In2), Divide18/2(In2), Divide23/2(In2), Divide9/2(In2)
  Add1_to_const/1 -> Divide6/1(In1)
  rsigma/1 -> Subtract/2(In2), Subtract1/2(In2), Subtract2/2(In2)

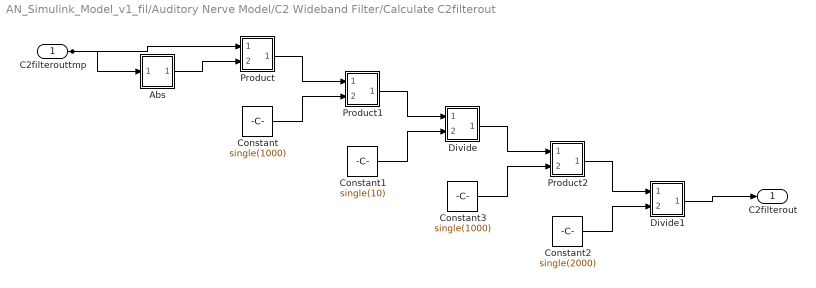
== system AN_Simulink_Model_v1_fil/Auditory Nerve Model/C2 Wideband Filter/Calculate C2filterout ==
  C2filterouttmp : Inport  OutDataTypeStr=single  PortDimensions=1  SampleTime=2.08333333333333e-05
  Abs : Subsystem
      mask Display: disp('NFP\nabs');
  Constant : Constant  Value=single(1000)  OutDataTypeStr=single  SampleTime=-1
  Constant1 : Constant  Value=single(10)  OutDataTypeStr=single  SampleTime=-1
  Constant2 : Constant  Value=single(2000)  OutDataTypeStr=single  SampleTime=-1
  Constant3 : Constant  Value=single(1000)  OutDataTypeStr=single  SampleTime=-1
  Divide : Subsystem
      mask Display: disp('NFP\nmul');
  Divide1 : Subsystem
      mask Display: disp('NFP\nmul');
  Product : Subsystem
      mask Display: disp('NFP\nmul');
  Product1 : Subsystem
      mask Display: disp('NFP\nmul');
  Product2 : Subsystem
      mask Display: disp('NFP\nmul');
  C2filterout : Outport  VectorParamsAs1DForOutWhenUnconnected=off
  wires:
  Product2/1(Out1) -> Divide1/1(In1)
  Product1/1(Out1) -> Divide/1(In1)
  Product/1(Out1) -> Product1/1(In1)
  Divide1/1(Out1) -> C2filterout/1
  Divide/1(Out1) -> Product2/1(In1)
  Abs/1(Out1) -> Product/2(In2)
  Constant3/1 -> Product2/2(In2)
  Constant2/1 -> Divide1/2(In2)
  Constant1/1 -> Divide/2(In2)
  Constant/1 -> Product1/2(In2)
  C2filterouttmp/1 -> Abs/1(In1), Product/1(In1)

== system AN_Simulink_Model_v1_fil/Auditory Nerve Model/C2 Wideband Filter/Gain ==
  In1 : Inport
  In2 : Inport  Port=2
  Gain : Product  Inputs=**  OutDataTypeStr=single  SampleTime=2.08333333333333e-05
  Out1 : Outport
  wires:
  Gain/1 -> Out1/1
  In2/1 -> Gain/2
  In1/1 -> Gain/1

== system AN_Simulink_Model_v1_fil/Auditory Nerve Model/C2 Wideband Filter/Gain10_unaryminus ==
  In1 : Inport
  Gain10_unaryminus : UnaryMinus  SampleTime=2.08333333333333e-05
  Out1 : Outport
  wires:
  Gain10_unaryminus/1 -> Out1/1
  In1/1 -> Gain10_unaryminus/1

== system AN_Simulink_Model_v1_fil/Auditory Nerve Model/C2 Wideband Filter/Gain1_unaryminus ==
  In1 : Inport
  Gain1_unaryminus : UnaryMinus  SampleTime=2.08333333333333e-05
  Out1 : Outport
  wires:
  Gain1_unaryminus/1 -> Out1/1
  In1/1 -> Gain1_unaryminus/1

== system AN_Simulink_Model_v1_fil/Auditory Nerve Model/C2 Wideband Filter/Gain2_unaryminus ==
  In1 : Inport
  Gain2_unaryminus : UnaryMinus  SampleTime=2.08333333333333e-05
  Out1 : Outport
  wires:
  Gain2_unaryminus/1 -> Out1/1
  In1/1 -> Gain2_unaryminus/1

== system AN_Simulink_Model_v1_fil/Auditory Nerve Model/C2 Wideband Filter/Gain3_unaryminus ==
  In1 : Inport
  Gain3_unaryminus : UnaryMinus  SampleTime=2.08333333333333e-05
  Out1 : Outport
  wires:
  Gain3_unaryminus/1 -> Out1/1
  In1/1 -> Gain3_unaryminus/1

== system AN_Simulink_Model_v1_fil/Auditory Nerve Model/C2 Wideband Filter/Gain4_unaryminus ==
  In1 : Inport
  Gain4_unaryminus : UnaryMinus  SampleTime=2.08333333333333e-05
  Out1 : Outport
  wires:
  Gain4_unaryminus/1 -> Out1/1
  In1/1 -> Gain4_unaryminus/1

== system AN_Simulink_Model_v1_fil/Auditory Nerve Model/C2 Wideband Filter/Gain5_unaryminus ==
  In1 : Inport
  Gain5_unaryminus : UnaryMinus  SampleTime=2.08333333333333e-05
  Out1 : Outport
  wires:
  Gain5_unaryminus/1 -> Out1/1
  In1/1 -> Gain5_unaryminus/1

== system AN_Simulink_Model_v1_fil/Auditory Nerve Model/C2 Wideband Filter/Gain6_unaryminus ==
  In1 : Inport
  Gain6_unaryminus : UnaryMinus  SampleTime=2.08333333333333e-05
  Out1 : Outport
  wires:
  Gain6_unaryminus/1 -> Out1/1
  In1/1 -> Gain6_unaryminus/1

== system AN_Simulink_Model_v1_fil/Auditory Nerve Model/C2 Wideband Filter/Gain7_unaryminus ==
  In1 : Inport
  Gain7_unaryminus : UnaryMinus  SampleTime=2.08333333333333e-05
  Out1 : Outport
  wires:
  Gain7_unaryminus/1 -> Out1/1
  In1/1 -> Gain7_unaryminus/1

== system AN_Simulink_Model_v1_fil/Auditory Nerve Model/C2 Wideband Filter/Gain8_unaryminus ==
  In1 : Inport
  Gain8_unaryminus : UnaryMinus  SampleTime=2.08333333333333e-05
  Out1 : Outport
  wires:
  Gain8_unaryminus/1 -> Out1/1
  In1/1 -> Gain8_unaryminus/1

== system AN_Simulink_Model_v1_fil/Auditory Nerve Model/C2 Wideband Filter/Gain9_unaryminus ==
  In1 : Inport
  Gain9_unaryminus : UnaryMinus  SampleTime=2.08333333333333e-05
  Out1 : Outport
  wires:
  Gain9_unaryminus/1 -> Out1/1
  In1/1 -> Gain9_unaryminus/1

== system AN_Simulink_Model_v1_fil/Auditory Nerve Model/C2 Wideband Filter/Product ==
  In1 : Inport
  In2 : Inport  Port=2
  Product : Product  Inputs=**  OutDataTypeStr=single  SampleTime=2.08333333333333e-05
  Out1 : Outport
  wires:
  Product/1 -> Out1/1
  In2/1 -> Product/2
  In1/1 -> Product/1

== system AN_Simulink_Model_v1_fil/Auditory Nerve Model/C2 Wideband Filter/Product1 ==
  In1 : Inport
  In2 : Inport  Port=2
  Product1 : Product  Inputs=**  OutDataTypeStr=single  SampleTime=2.08333333333333e-05
  Out1 : Outport
  wires:
  Product1/1 -> Out1/1
  In2/1 -> Product1/2
  In1/1 -> Product1/1

== system AN_Simulink_Model_v1_fil/Auditory Nerve Model/C2 Wideband Filter/Product10 ==
  In1 : Inport
  In2 : Inport  Port=2
  Product10 : Product  Inputs=**  OutDataTypeStr=single  SampleTime=2.08333333333333e-05
  Out1 : Outport
  wires:
  Product10/1 -> Out1/1
  In2/1 -> Product10/2
  In1/1 -> Product10/1

== system AN_Simulink_Model_v1_fil/Auditory Nerve Model/C2 Wideband Filter/Product11 ==
  In1 : Inport
  In2 : Inport  Port=2
  Product11 : Product  Inputs=**  OutDataTypeStr=single  SampleTime=2.08333333333333e-05
  Out1 : Outport
  wires:
  Product11/1 -> Out1/1
  In2/1 -> Product11/2
  In1/1 -> Product11/1

== system AN_Simulink_Model_v1_fil/Auditory Nerve Model/C2 Wideband Filter/Product12 ==
  In1 : Inport
  In2 : Inport  Port=2
  Product12 : Product  Inputs=**  OutDataTypeStr=single  SampleTime=2.08333333333333e-05
  Out1 : Outport
  wires:
  Product12/1 -> Out1/1
  In2/1 -> Product12/2
  In1/1 -> Product12/1

== system AN_Simulink_Model_v1_fil/Auditory Nerve Model/C2 Wideband Filter/Product13 ==
  In1 : Inport
  In2 : Inport  Port=2
  Product13 : Product  Inputs=**  OutDataTypeStr=single  SampleTime=2.08333333333333e-05
  Out1 : Outport
  wires:
  Product13/1 -> Out1/1
  In2/1 -> Product13/2
  In1/1 -> Product13/1

== system AN_Simulink_Model_v1_fil/Auditory Nerve Model/C2 Wideband Filter/Product14 ==
  In1 : Inport
  In2 : Inport  Port=2
  Product14 : Product  Inputs=**  OutDataTypeStr=single  SampleTime=2.08333333333333e-05
  Out1 : Outport
  wires:
  Product14/1 -> Out1/1
  In2/1 -> Product14/2
  In1/1 -> Product14/1

== system AN_Simulink_Model_v1_fil/Auditory Nerve Model/C2 Wideband Filter/Product15 ==
  In1 : Inport
  In2 : Inport  Port=2
  Product15 : Product  Inputs=**  OutDataTypeStr=single  SampleTime=2.08333333333333e-05
  Out1 : Outport
  wires:
  Product15/1 -> Out1/1
  In2/1 -> Product15/2
  In1/1 -> Product15/1

== system AN_Simulink_Model_v1_fil/Auditory Nerve Model/C2 Wideband Filter/Product16 ==
  In1 : Inport
  In2 : Inport  Port=2
  Product16 : Product  Inputs=**  OutDataTypeStr=single  SampleTime=2.08333333333333e-05
  Out1 : Outport
  wires:
  Product16/1 -> Out1/1
  In2/1 -> Product16/2
  In1/1 -> Product16/1

== system AN_Simulink_Model_v1_fil/Auditory Nerve Model/C2 Wideband Filter/Product17 ==
  In1 : Inport
  In2 : Inport  Port=2
  Product17 : Product  Inputs=**  OutDataTypeStr=single  SampleTime=2.08333333333333e-05
  Out1 : Outport
  wires:
  Product17/1 -> Out1/1
  In2/1 -> Product17/2
  In1/1 -> Product17/1

== system AN_Simulink_Model_v1_fil/Auditory Nerve Model/C2 Wideband Filter/Product18 ==
  In1 : Inport
  In2 : Inport  Port=2
  Product18 : Product  Inputs=**  OutDataTypeStr=single  SampleTime=2.08333333333333e-05
  Out1 : Outport
  wires:
  Product18/1 -> Out1/1
  In2/1 -> Product18/2
  In1/1 -> Product18/1

== system AN_Simulink_Model_v1_fil/Auditory Nerve Model/C2 Wideband Filter/Product19 ==
  In1 : Inport
  In2 : Inport  Port=2
  Product19 : Product  Inputs=**  OutDataTypeStr=single  SampleTime=2.08333333333333e-05
  Out1 : Outport
  wires:
  Product19/1 -> Out1/1
  In2/1 -> Product19/2
  In1/1 -> Product19/1

== system AN_Simulink_Model_v1_fil/Auditory Nerve Model/C2 Wideband Filter/Product2 ==
  In1 : Inport
  In2 : Inport  Port=2
  Product2 : Product  Inputs=**  OutDataTypeStr=single  SampleTime=2.08333333333333e-05
  Out1 : Outport
  wires:
  Product2/1 -> Out1/1
  In2/1 -> Product2/2
  In1/1 -> Product2/1

== system AN_Simulink_Model_v1_fil/Auditory Nerve Model/C2 Wideband Filter/Product20 ==
  In1 : Inport
  In2 : Inport  Port=2
  Product20 : Product  Inputs=**  OutDataTypeStr=single  SampleTime=2.08333333333333e-05
  Out1 : Outport
  wires:
  Product20/1 -> Out1/1
  In2/1 -> Product20/2
  In1/1 -> Product20/1

== system AN_Simulink_Model_v1_fil/Auditory Nerve Model/C2 Wideband Filter/Product21 ==
  In1 : Inport
  In2 : Inport  Port=2
  Product21 : Product  Inputs=**  OutDataTypeStr=single  SampleTime=2.08333333333333e-05
  Out1 : Outport
  wires:
  Product21/1 -> Out1/1
  In2/1 -> Product21/2
  In1/1 -> Product21/1

== system AN_Simulink_Model_v1_fil/Auditory Nerve Model/C2 Wideband Filter/Product22 ==
  In1 : Inport
  In2 : Inport  Port=2
  Product22 : Product  Inputs=**  OutDataTypeStr=single  SampleTime=2.08333333333333e-05
  Out1 : Outport
  wires:
  Product22/1 -> Out1/1
  In2/1 -> Product22/2
  In1/1 -> Product22/1

== system AN_Simulink_Model_v1_fil/Auditory Nerve Model/C2 Wideband Filter/Product23 ==
  In1 : Inport
  In2 : Inport  Port=2
  Product23 : Product  Inputs=**  OutDataTypeStr=single  SampleTime=2.08333333333333e-05
  Out1 : Outport
  wires:
  Product23/1 -> Out1/1
  In2/1 -> Product23/2
  In1/1 -> Product23/1

== system AN_Simulink_Model_v1_fil/Auditory Nerve Model/C2 Wideband Filter/Product24 ==
  In1 : Inport
  In2 : Inport  Port=2
  Product24 : Product  Inputs=**  OutDataTypeStr=single  SampleTime=2.08333333333333e-05
  Out1 : Outport
  wires:
  Product24/1 -> Out1/1
  In2/1 -> Product24/2
  In1/1 -> Product24/1

== system AN_Simulink_Model_v1_fil/Auditory Nerve Model/C2 Wideband Filter/Product3 ==
  In1 : Inport
  In2 : Inport  Port=2
  Product3 : Product  Inputs=**  OutDataTypeStr=single  SampleTime=2.08333333333333e-05
  Out1 : Outport
  wires:
  Product3/1 -> Out1/1
  In2/1 -> Product3/2
  In1/1 -> Product3/1

== system AN_Simulink_Model_v1_fil/Auditory Nerve Model/C2 Wideband Filter/Product4 ==
  In1 : Inport
  In2 : Inport  Port=2
  Product4 : Product  Inputs=**  OutDataTypeStr=single  SampleTime=2.08333333333333e-05
  Out1 : Outport
  wires:
  Product4/1 -> Out1/1
  In2/1 -> Product4/2
  In1/1 -> Product4/1

== system AN_Simulink_Model_v1_fil/Auditory Nerve Model/C2 Wideband Filter/Product5 ==
  In1 : Inport
  In2 : Inport  Port=2
  Product5 : Product  Inputs=**  OutDataTypeStr=single  SampleTime=2.08333333333333e-05
  Out1 : Outport
  wires:
  Product5/1 -> Out1/1
  In2/1 -> Product5/2
  In1/1 -> Product5/1

== system AN_Simulink_Model_v1_fil/Auditory Nerve Model/C2 Wideband Filter/Product6 ==
  In1 : Inport
  In2 : Inport  Port=2
  Product6 : Product  Inputs=**  OutDataTypeStr=single  SampleTime=2.08333333333333e-05
  Out1 : Outport
  wires:
  Product6/1 -> Out1/1
  In2/1 -> Product6/2
  In1/1 -> Product6/1

== system AN_Simulink_Model_v1_fil/Auditory Nerve Model/C2 Wideband Filter/Product7 ==
  In1 : Inport
  In2 : Inport  Port=2
  Product7 : Product  Inputs=**  OutDataTypeStr=single  SampleTime=2.08333333333333e-05
  Out1 : Outport
  wires:
  Product7/1 -> Out1/1
  In2/1 -> Product7/2
  In1/1 -> Product7/1

== system AN_Simulink_Model_v1_fil/Auditory Nerve Model/C2 Wideband Filter/Product8 ==
  In1 : Inport
  In2 : Inport  Port=2
  Product8 : Product  Inputs=**  OutDataTypeStr=single  SampleTime=2.08333333333333e-05
  Out1 : Outport
  wires:
  Product8/1 -> Out1/1
  In2/1 -> Product8/2
  In1/1 -> Product8/1

== system AN_Simulink_Model_v1_fil/Auditory Nerve Model/C2 Wideband Filter/Product9 ==
  In1 : Inport
  In2 : Inport  Port=2
  Product9 : Product  Inputs=**  OutDataTypeStr=single  SampleTime=2.08333333333333e-05
  Out1 : Outport
  wires:
  Product9/1 -> Out1/1
  In2/1 -> Product9/2
  In1/1 -> Product9/1

== system AN_Simulink_Model_v1_fil/Auditory Nerve Model/C2 Wideband Filter/Sum ==
  In1 : Inport
  In2 : Inport  Port=2
  Sum : Sum  OutDataTypeStr=single  SampleTime=2.08333333333333e-05  SaturateOnIntegerOverflow=on  InputSameDT=on
  Out1 : Outport
  wires:
  Sum/1 -> Out1/1
  In2/1 -> Sum/2
  In1/1 -> Sum/1

== system AN_Simulink_Model_v1_fil/Auditory Nerve Model/C2 Wideband Filter/Sum1 ==
  In1 : Inport
  In2 : Inport  Port=2
  Sum1 : Sum  OutDataTypeStr=single  SampleTime=2.08333333333333e-05  SaturateOnIntegerOverflow=on  InputSameDT=on
  Out1 : Outport
  wires:
  Sum1/1 -> Out1/1
  In2/1 -> Sum1/2
  In1/1 -> Sum1/1

== system AN_Simulink_Model_v1_fil/Auditory Nerve Model/C2 Wideband Filter/Sum10 ==
  In1 : Inport
  In2 : Inport  Port=2
  Sum10 : Sum  OutDataTypeStr=single  SampleTime=2.08333333333333e-05  SaturateOnIntegerOverflow=on  InputSameDT=on
  Out1 : Outport
  wires:
  Sum10/1 -> Out1/1
  In2/1 -> Sum10/2
  In1/1 -> Sum10/1

== system AN_Simulink_Model_v1_fil/Auditory Nerve Model/C2 Wideband Filter/Sum11 ==
  In1 : Inport
  In2 : Inport  Port=2
  Sum11 : Sum  OutDataTypeStr=single  SampleTime=2.08333333333333e-05  SaturateOnIntegerOverflow=on  InputSameDT=on
  Out1 : Outport
  wires:
  Sum11/1 -> Out1/1
  In2/1 -> Sum11/2
  In1/1 -> Sum11/1

== system AN_Simulink_Model_v1_fil/Auditory Nerve Model/C2 Wideband Filter/Sum12 ==
  In1 : Inport
  In2 : Inport  Port=2
  Sum12 : Sum  OutDataTypeStr=single  SampleTime=2.08333333333333e-05  SaturateOnIntegerOverflow=on  InputSameDT=on
  Out1 : Outport
  wires:
  Sum12/1 -> Out1/1
  In2/1 -> Sum12/2
  In1/1 -> Sum12/1

== system AN_Simulink_Model_v1_fil/Auditory Nerve Model/C2 Wideband Filter/Sum13 ==
  In1 : Inport
  In2 : Inport  Port=2
  Sum13 : Sum  OutDataTypeStr=single  SampleTime=2.08333333333333e-05  SaturateOnIntegerOverflow=on  InputSameDT=on
  Out1 : Outport
  wires:
  Sum13/1 -> Out1/1
  In2/1 -> Sum13/2
  In1/1 -> Sum13/1

== system AN_Simulink_Model_v1_fil/Auditory Nerve Model/C2 Wideband Filter/Sum14 ==
  In1 : Inport
  In2 : Inport  Port=2
  Sum14 : Sum  OutDataTypeStr=single  SampleTime=2.08333333333333e-05  SaturateOnIntegerOverflow=on  InputSameDT=on
  Out1 : Outport
  wires:
  Sum14/1 -> Out1/1
  In2/1 -> Sum14/2
  In1/1 -> Sum14/1

== system AN_Simulink_Model_v1_fil/Auditory Nerve Model/C2 Wideband Filter/Sum15 ==
  In1 : Inport
  In2 : Inport  Port=2
  Sum15 : Sum  OutDataTypeStr=single  SampleTime=2.08333333333333e-05  SaturateOnIntegerOverflow=on  InputSameDT=on
  Out1 : Outport
  wires:
  Sum15/1 -> Out1/1
  In2/1 -> Sum15/2
  In1/1 -> Sum15/1

== system AN_Simulink_Model_v1_fil/Auditory Nerve Model/C2 Wideband Filter/Sum16 ==
  In1 : Inport
  In2 : Inport  Port=2
  Sum16 : Sum  OutDataTypeStr=single  SampleTime=2.08333333333333e-05  SaturateOnIntegerOverflow=on  InputSameDT=on
  Out1 : Outport
  wires:
  Sum16/1 -> Out1/1
  In2/1 -> Sum16/2
  In1/1 -> Sum16/1

== system AN_Simulink_Model_v1_fil/Auditory Nerve Model/C2 Wideband Filter/Sum17 ==
  In1 : Inport
  In2 : Inport  Port=2
  Sum17 : Sum  OutDataTypeStr=single  SampleTime=2.08333333333333e-05  SaturateOnIntegerOverflow=on  InputSameDT=on
  Out1 : Outport
  wires:
  Sum17/1 -> Out1/1
  In2/1 -> Sum17/2
  In1/1 -> Sum17/1

== system AN_Simulink_Model_v1_fil/Auditory Nerve Model/C2 Wideband Filter/Sum18 ==
  In1 : Inport
  In2 : Inport  Port=2
  Sum18 : Sum  OutDataTypeStr=single  SampleTime=2.08333333333333e-05  SaturateOnIntegerOverflow=on  InputSameDT=on
  Out1 : Outport
  wires:
  Sum18/1 -> Out1/1
  In2/1 -> Sum18/2
  In1/1 -> Sum18/1

== system AN_Simulink_Model_v1_fil/Auditory Nerve Model/C2 Wideband Filter/Sum19 ==
  In1 : Inport
  In2 : Inport  Port=2
  Sum19 : Sum  OutDataTypeStr=single  SampleTime=2.08333333333333e-05  SaturateOnIntegerOverflow=on  InputSameDT=on
  Out1 : Outport
  wires:
  Sum19/1 -> Out1/1
  In2/1 -> Sum19/2
  In1/1 -> Sum19/1

== system AN_Simulink_Model_v1_fil/Auditory Nerve Model/C2 Wideband Filter/Sum2 ==
  In1 : Inport
  In2 : Inport  Port=2
  Sum2 : Sum  OutDataTypeStr=single  SampleTime=2.08333333333333e-05  SaturateOnIntegerOverflow=on  InputSameDT=on
  Out1 : Outport
  wires:
  Sum2/1 -> Out1/1
  In2/1 -> Sum2/2
  In1/1 -> Sum2/1

== system AN_Simulink_Model_v1_fil/Auditory Nerve Model/C2 Wideband Filter/Sum3 ==
  In1 : Inport
  In2 : Inport  Port=2
  Sum3 : Sum  OutDataTypeStr=single  SampleTime=2.08333333333333e-05  SaturateOnIntegerOverflow=on  InputSameDT=on
  Out1 : Outport
  wires:
  Sum3/1 -> Out1/1
  In2/1 -> Sum3/2
  In1/1 -> Sum3/1

== system AN_Simulink_Model_v1_fil/Auditory Nerve Model/C2 Wideband Filter/Sum4 ==
  In1 : Inport
  In2 : Inport  Port=2
  Sum4 : Sum  OutDataTypeStr=single  SampleTime=2.08333333333333e-05  SaturateOnIntegerOverflow=on  InputSameDT=on
  Out1 : Outport
  wires:
  Sum4/1 -> Out1/1
  In2/1 -> Sum4/2
  In1/1 -> Sum4/1

== system AN_Simulink_Model_v1_fil/Auditory Nerve Model/C2 Wideband Filter/Sum5 ==
  In1 : Inport
  In2 : Inport  Port=2
  Sum5 : Sum  OutDataTypeStr=single  SampleTime=2.08333333333333e-05  SaturateOnIntegerOverflow=on  InputSameDT=on
  Out1 : Outport
  wires:
  Sum5/1 -> Out1/1
  In2/1 -> Sum5/2
  In1/1 -> Sum5/1

== system AN_Simulink_Model_v1_fil/Auditory Nerve Model/C2 Wideband Filter/Sum6 ==
  In1 : Inport
  In2 : Inport  Port=2
  Sum6 : Sum  OutDataTypeStr=single  SampleTime=2.08333333333333e-05  SaturateOnIntegerOverflow=on  InputSameDT=on
  Out1 : Outport
  wires:
  Sum6/1 -> Out1/1
  In2/1 -> Sum6/2
  In1/1 -> Sum6/1
